simulink model "Pendulum"  (R2021b)
settings: Solver=VariableStepAuto  StartTime=0.0  StopTime=10.0  RelTol=1e-3
values from neighbouring files (symbols this model uses):
  b = 0.1    [VariablesDelSistema.m]
  g = -9.81    [VariablesDelSistema.m]
  I = 0.006    [VariablesDelSistema.m]
  L = 0.5 + 0.1*8    (= 1.3)    [VariablesDelSistema.m]
  m = 0.2    [VariablesDelSistema.m]
  M = 0.5 + 0.1*7    (= 1.2)    [VariablesDelSistema.m]
settings Model: Creator=jualc  LastModifiedBy=e.delpico.2020

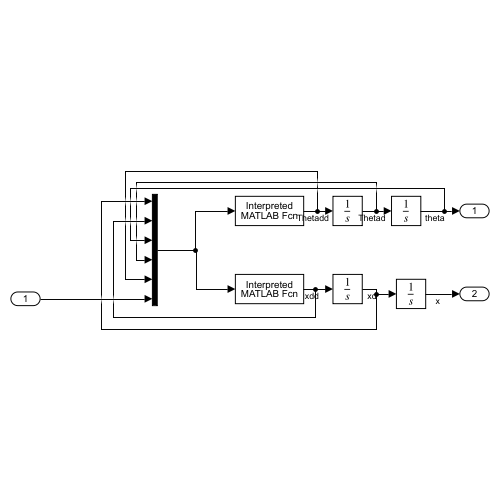
[thumbnail: Simulink's stored preview of the top-level diagram]
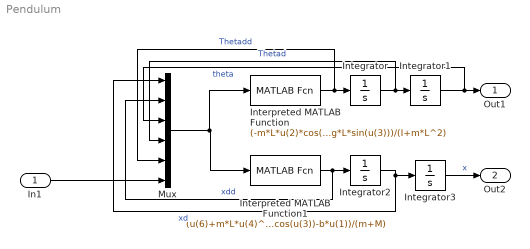
== system Pendulum ==
  In1 : Inport
  Integrator : Integrator
  Integrator1 : Integrator  InitialCondition=pi
  Integrator2 : Integrator
  Integrator3 : Integrator  InitialCondition=pi
  Interpreted MATLAB Function : MATLABFcn  MATLABFcn=(-m*L*u(2)*cos(u(3))-m*g*L*sin(u(3)))/(I+m*L^2)
  Interpreted MATLAB Function1 : MATLABFcn  MATLABFcn=(u(6)+m*L*u(4)^2*sin(u(3))-m*L*u(5)*cos(u(3))-b*u(1))/(m+M)
  Mux : Mux  Inputs=6
  Out1 : Outport
  Out2 : Outport  Port=2
  wires:
  In1/1 -> Mux/6
  Mux/1 -> Interpreted MATLAB Function/1, Interpreted MATLAB Function1/1
  Interpreted MATLAB Function/1 -> Mux/5, Integrator/1  "Thetadd"
  Interpreted MATLAB Function1/1 -> Mux/2, Integrator2/1  "xdd"
  Integrator2/1 -> Integrator3/1, Mux/1  "xd"
  Integrator/1 -> Mux/4, Integrator1/1  "Thetad"
  Integrator1/1 -> Out1/1, Mux/3  "theta"
  Integrator3/1 -> Out2/1  "x"
